simulink model "feedback_linearization_control"  (R2019a)
settings: Solver=FixedStepAuto  StartTime=0.0  StopTime=3  FixedStep=0.01  RelTol=1e-3
settings Model: Creator=Shayan  LastModifiedBy=bikra
settings DataIOCC: ReturnWorkspaceOutputs=off
settings OptimizationCC: LifeSpan=inf
settings DebuggingCC: ArithmeticOperatorsInVariantConditions=warning
settings CodeAppCC: StateflowObjectComments=on

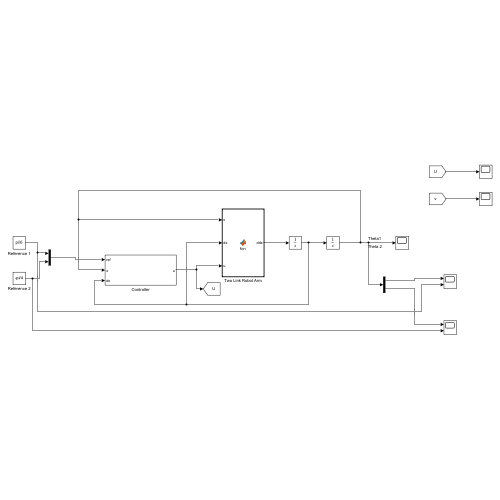
[thumbnail: Simulink's stored preview of the top-level diagram]
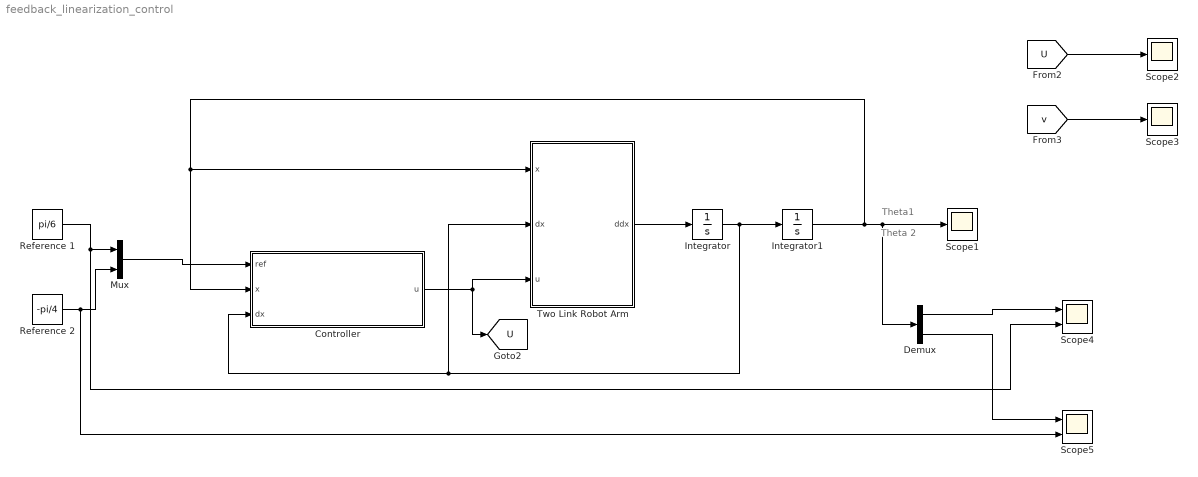
== system feedback_linearization_control ==
  note: Theta 2
  note: Theta1
  Controller : Subsystem
  Demux : Demux  Outputs=2
  Integrator : Integrator  InitialCondition=[0 0]
  Integrator1 : Integrator  InitialCondition=[pi/2 pi/2]
  Mux : Mux  Inputs=2
  Reference 1 : Constant  Value=pi/6
  Reference 2 : Constant  Value=-pi/4
  Scope1 : Scope
  Scope2 : Scope
  Scope3 : Scope
  Scope4 : Scope  NumInputPorts=2
  Scope5 : Scope  NumInputPorts=2
  Two Link Robot Arm : MATLAB Function  TreatAsAtomicUnit=on
  tag scope: U=global
  wires:
  Integrator/1 -> Two Link Robot Arm/2(dx), Controller/3(dx), Integrator1/1
  Two Link Robot Arm/1(ddx) -> Integrator/1
  Integrator1/1 -> Two Link Robot Arm/1(x), Controller/2(x), Demux/1, Scope1/1
  Mux/1 -> Controller/1(ref)
  Controller/1(u) -> Two Link Robot Arm/3(u), [U]
  [U] -> Scope2/1
  [v] -> Scope3/1
  Reference 1/1 -> Mux/1, Scope4/2
  Reference 2/1 -> Mux/2, Scope5/2
  Demux/1 -> Scope4/1
  Demux/2 -> Scope5/1

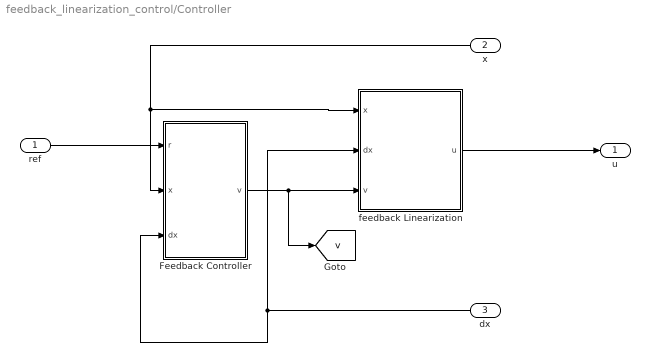
== system feedback_linearization_control/Controller ==
  ref : Inport
  x : Inport  Port=2
  dx : Inport  Port=3
  Feedback Controller : MATLAB Function  TreatAsAtomicUnit=on
  feedback Linearization : MATLAB Function  TreatAsAtomicUnit=on
  u : Outport
  tag scope: v=global
  wires:
  ref/1 -> Feedback Controller/1(r)
  x/1 -> feedback Linearization/1(x), Feedback Controller/2(x)
  Feedback Controller/1(v) -> [v], feedback Linearization/3(v)
  dx/1 -> feedback Linearization/2(dx), Feedback Controller/3(dx)
  feedback Linearization/1(u) -> u/1

== matlab function feedback_linearization_control/Controller/feedback Linearization ==
  data: x input; dx input; u output; v input
function u = fcn(x,dx,v)

M1 = 1;
M2 = 1;
L1 = 2;
L2 = 1;
g = 9.81;

G = [(M1+M2)*g*L1*cos(x(1));
    M2*g*L2*cos(x(2))];
C = [M2*L1*L2*(dx(2)^2)*sin(x(1)-x(2));
    -M2*L1*L2*(dx(1)^2)*sin(x(1)-x(2))];
M = [(M1+M2)*L1^2, M2*L1*L2*cos(x(1)-x(2));
     M2*L1*L2*cos(x(1)-x(2)),  M2*L2^2;];


u = M*v + C + G;

== matlab function feedback_linearization_control/Two Link Robot Arm ==
  data: x input; dx input; u input; ddx output
function ddx = fcn(x,dx,u)

M1 = 1;
M2 = 1;
L1 = 2;
L2 = 1;
g = 9.81;
G = [(M1+M2)*g*L1*cos(x(1));
    M2*g*L2*cos(x(2))];
C = [M2*L1*L2*(dx(2)^2)*sin(x(1)-x(2));
    -M2*L1*L2*(dx(1)^2)*sin(x(1)-x(2))];
M = [(M1+M2)*L1^2, M2*L1*L2*cos(x(1)-x(2));
     M2*L1*L2*cos(x(1)-x(2)),  M2*L2^2;];
ddx = inv(M)*(-C-G+u);

== matlab function feedback_linearization_control/Controller/Feedback Controller ==
  data: r input; v output; x input; dx input
function v  = fcn(r,x,dx)

k1 = 15.99;
k2 = 5.65;
k3 = k1;

v = [k3*r(1) - k1*x(1) - k2*dx(1);...
     (k3*r(2) - k1*x(2) - k2*dx(2));];
